simulink model "CoupledTanks_original"  (R2023b)
settings: Solver=ode45  StartTime=0.0  StopTime=400  MaxStep=1e-1  RelTol=1e-3  EnableMultiTasking=on
InitFcn:
  | g = 9.81; %gravitational constant
  | 
  | % showVR = 1; %show VR world
  | % h1_init = 0; %initial condition
  | % h2_init = 0; %initial condition
values from neighbouring files (symbols this model uses):
  K = place(Acl,Bcl, xd)    [ARI_SEM.m]
undefined symbols (not defined in the file or in its folder): P
libraries: vrlib x56, cstblocks x3, slpidlib x1
(part 1 of 2)
CloseFcn:
  | vrclose all;
  | clear figureVR worldVR;
settings Model: Creator=H  LastModifiedBy=pinki
settings SolverCC: AlgebraicLoopSolver=TrustRegion
settings DataIOCC: LimitDataPoints=on  SaveFormat=Array  SignalLoggingSaveFormat=ModelDataLogs  ReturnWorkspaceOutputs=off
settings OptimizationCC: ExpressionDepthLimit=2147483647  InitFltsAndDblsToZero=on  LifeSpan=inf
settings DebuggingCC: SaveWithParameterizedLinksMsg=none  UnderspecifiedInitializationDetection=Classic  MergeDetectMultiDrivingBlocksExec=none  SignalResolutionControl=TryResolveAllWithWarning  SolverPrmCheckMsg=warning  FcnCallInpInsideContextMsg=warning  UnconnectedInputMsg=warning  UnconnectedOutputMsg=warning  UnconnectedLineMsg=warning  StateNameClashWarn=warning  SFUnexpectedBacktrackingDiag=warning  SFNoUnconditionalDefaultTransitionDiag=warning  SFExecutionAtInitializationDiag=none  ArithmeticOperatorsInVariantConditions=warning
settings HardwareCC: ProdBitPerPointer=32  ProdBitPerSizeT=32  ProdBitPerPtrDiffT=32  ProdLargestAtomicFloat=None  ProdIntDivRoundTo=Undefined  ProdEndianess=Unspecified  ProdWordSize=32  ProdHWDeviceType=32-bit Generic
settings ModelReferenceCC: PropagateSignalLabelsOutOfModel=off
settings SFSimCC: SimUseLocalCustomCode=off  CustomCodeUndefinedFunction=UseInterfaceOnly
settings RTWCC: RTWUseLocalCustomCode=off
settings CodeAppCC: StateflowObjectComments=on
settings GRTTargetCC: TargetFcnLib=ansi_tfl_tmw.mat  TargetLangStandard=C89/C90 (ANSI)  CombineOutputUpdateFcns=off  GRTInterface=on
settings ConfigComp: CovMetricSettings=dw  CovSaveCumulativeToWorkspaceVar=on  CovSaveSingleToWorkspaceVar=on  CovExternalEMLEnable=off

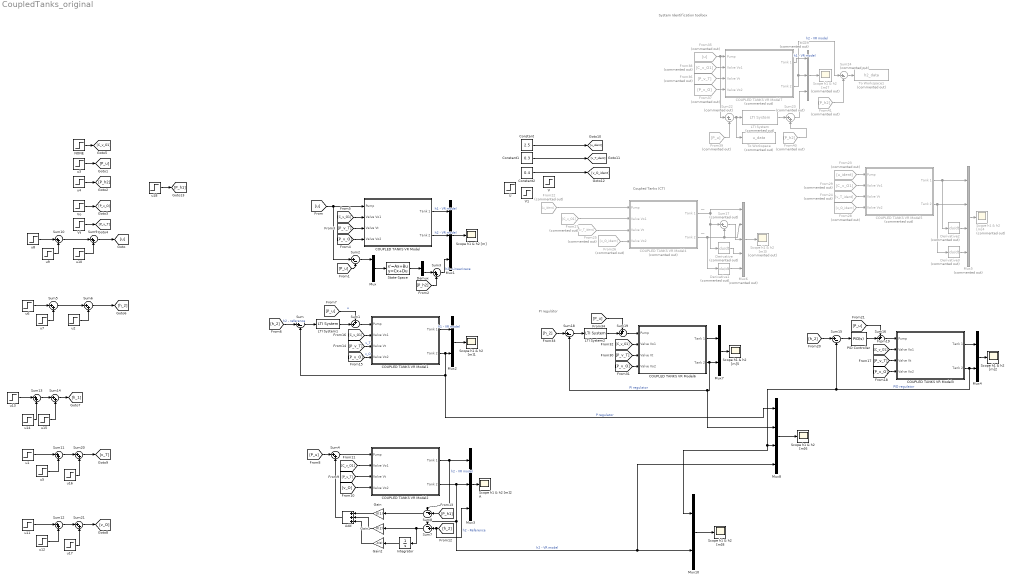
== system CoupledTanks_original ==
  note: System Identification toolbox
  note: PI regulátor
  note: __
  note: Coupled Tanks (CT)
  note: __
  Add : Sum  Inputs=+++
  COUPLED TANKS VR Model : Subsystem  mask(Coupled Tanks (CT) in laboratory K26){showVR=off, sfcnParam1=P.h1, sfcnParam2=P.h2}
      mask prompts: showVR "Show VirtualWorld?"; sfcnParam1 "Initial fluid level in the left tank 1   h1(0)  [cm]"; sfcnParam2 "Initial fluid  level in the right tank 2   h2 (0) [cm]"
      mask help:
      | Coupled Tanks (CT) in laboratory K26 - Virtual Reality
      | Real-Time Workshop generated S-function.
      mask Help:
      | Couple Tanks in laboratory K26 - Virtual Reality. <br><br>
      | 
      | 
      | This is a&nbsp;virtual model of the Coupled Tanks apparatus in Laboratory of automatic control
      | theory&nbsp;26 (<a href="http://support.dce.felk.cvut.cz/lab26/" target="_blank">http://support.dce.felk.cvut.cz/lab26/</a>),
      | which consists of a&nbsp;gear-pump, two tanks (left and right), inflow and outflow pipes and transfer (V<sub>t</sub>) and
      | output valves (V<sub>o1</sub>, V<sub>o2</sub>). The&nbsp;left tank is filled with the&nbsp;fluid by the&nbsp;gear-pump
      | controller by the&nbsp;voltage&nbsp;<em>u</em>&nbsp;[V]. The&nbsp;fluid can drain from the&nbsp;left tank through
      | the&nbsp;valve&nbsp;<em>v</em><sub>o1</sub>&nbsp;[%] or can drain to the&nbsp;right tank through the&nbsp;transfer
      | valve&nbsp;<em>v</em><sub>t</sub>&nbsp;[%]. The&nbsp;fluid drains away from the&nbsp;right tank through
      | the&nbsp;valve&nbsp;<em>v</em><sub>o2</sub>&nbsp;[%].<br><br>
      | 
      | The&nbsp;system input are the&nbsp;voltage of the&nbsp;motor of the&nbsp;gear-pump&nbsp;<em>u</em>&nbsp;[V]
      | and the&nbsp;opening of
      | the&nbsp;valves&nbsp;<em>v</em><sub>o1</sub>,&nbsp;<em>v</em><sub>t</sub>,&nbsp;<em>v</em><sub>o2</sub>&nbsp;[%].
      | The&nbsp;system outputs are the&nbsp;levels of the&nbsp;fluid in
      | the&nbsp;tanks&nbsp;<em>h</em><sub>1</sub>,&nbsp;<em>h</em><sub>2</sub>&nbsp;[cm].
      | The&nbsp;dynamics of the&nbsp;gear-pump is neglected. More information can be found on the&nbsp;website
      | <a href="http://support.dce.felk.cvut.cz/lab26/" target="_blank">http://support.dce.felk.cvut.cz/lab26/</a>.<br><br>
      | 
      | 
      | In the mask of the model, it can be set:
      | <ul>
      | <li>Initial fluid level in the left tank</li>
      | <li>Initial fluid level in the right tank.</li>
      | </ul><br><br>
      | 
      | 
      | Copyright: 2008, Jan Kricka, Jirka Roubal, Petr Husek.
      mask Callback showVR:
      | if strcmp('off',get_param(gcb,'showVR'))
      |     vrclose all;
      | else
      |     if exist('figureVR')==0
      |         figureVR = vrfigure;
      |     end
      |     if exist('worldVR')==0
      |         worldVR = vrworld('CoupledTanks_VR.WRL');
      |     end
      | 	if isvalid(figureVR)==0
      |         open(worldVR);
      |         figureVR = vrfigure(worldVR,[650 80 550 350]);
      | 	end
      | end
      mask Display:
      | image(imread('CoupledTanks_Image.jpg'));
      | port_label ('input',1,'u [V]');
      | port_label ('input',2,'Vo1 [-]');
      | port_label ('input',3,'Vt [-]');
      | port_label ('input',4,'Vo2 [-]');
      | port_label ('output',1,'h1 [m]');
      | port_label ('output',2,'h2 [m]');
  COUPLED TANKS VR Model1 : Subsystem  mask(Coupled Tanks (CT) in laboratory K26){showVR=off, sfcnParam1=P.h1, sfcnParam2=P.h2}
      mask prompts: showVR "Show VirtualWorld?"; sfcnParam1 "Initial fluid level in the left tank 1   h1(0)  [cm]"; sfcnParam2 "Initial fluid  level in the right tank 2   h2 (0) [cm]"
      mask help:
      | Coupled Tanks (CT) in laboratory K26 - Virtual Reality
      | Real-Time Workshop generated S-function.
      mask Help:
      | Couple Tanks in laboratory K26 - Virtual Reality. <br><br>
      | 
      | 
      | This is a&nbsp;virtual model of the Coupled Tanks apparatus in Laboratory of automatic control
      | theory&nbsp;26 (<a href="http://support.dce.felk.cvut.cz/lab26/" target="_blank">http://support.dce.felk.cvut.cz/lab26/</a>),
      | which consists of a&nbsp;gear-pump, two tanks (left and right), inflow and outflow pipes and transfer (V<sub>t</sub>) and
      | output valves (V<sub>o1</sub>, V<sub>o2</sub>). The&nbsp;left tank is filled with the&nbsp;fluid by the&nbsp;gear-pump
      | controller by the&nbsp;voltage&nbsp;<em>u</em>&nbsp;[V]. The&nbsp;fluid can drain from the&nbsp;left tank through
      | the&nbsp;valve&nbsp;<em>v</em><sub>o1</sub>&nbsp;[%] or can drain to the&nbsp;right tank through the&nbsp;transfer
      | valve&nbsp;<em>v</em><sub>t</sub>&nbsp;[%]. The&nbsp;fluid drains away from the&nbsp;right tank through
      | the&nbsp;valve&nbsp;<em>v</em><sub>o2</sub>&nbsp;[%].<br><br>
      | 
      | The&nbsp;system input are the&nbsp;voltage of the&nbsp;motor of the&nbsp;gear-pump&nbsp;<em>u</em>&nbsp;[V]
      | and the&nbsp;opening of
      | the&nbsp;valves&nbsp;<em>v</em><sub>o1</sub>,&nbsp;<em>v</em><sub>t</sub>,&nbsp;<em>v</em><sub>o2</sub>&nbsp;[%].
      | The&nbsp;system outputs are the&nbsp;levels of the&nbsp;fluid in
      | the&nbsp;tanks&nbsp;<em>h</em><sub>1</sub>,&nbsp;<em>h</em><sub>2</sub>&nbsp;[cm].
      | The&nbsp;dynamics of the&nbsp;gear-pump is neglected. More information can be found on the&nbsp;website
      | <a href="http://support.dce.felk.cvut.cz/lab26/" target="_blank">http://support.dce.felk.cvut.cz/lab26/</a>.<br><br>
      | 
      | 
      | In the mask of the model, it can be set:
      | <ul>
      | <li>Initial fluid level in the left tank</li>
      | <li>Initial fluid level in the right tank.</li>
      | </ul><br><br>
      | 
      | 
      | Copyright: 2008, Jan Kricka, Jirka Roubal, Petr Husek.
      mask Callback showVR:
      | if strcmp('off',get_param(gcb,'showVR'))
      |     vrclose all;
      | else
      |     if exist('figureVR')==0
      |         figureVR = vrfigure;
      |     end
      |     if exist('worldVR')==0
      |         worldVR = vrworld('CoupledTanks_VR.WRL');
      |     end
      | 	if isvalid(figureVR)==0
      |         open(worldVR);
      |         figureVR = vrfigure(worldVR,[650 80 550 350]);
      | 	end
      | end
      mask Display:
      | image(imread('CoupledTanks_Image.jpg'));
      | port_label ('input',1,'u [V]');
      | port_label ('input',2,'Vo1 [-]');
      | port_label ('input',3,'Vt [-]');
      | port_label ('input',4,'Vo2 [-]');
      | port_label ('output',1,'h1 [m]');
      | port_label ('output',2,'h2 [m]');
  COUPLED TANKS VR Model2 : Subsystem  mask(Coupled Tanks (CT) in laboratory K26){showVR=off, sfcnParam1=P.h1, sfcnParam2=P.h2}
      mask prompts: showVR "Show VirtualWorld?"; sfcnParam1 "Initial fluid level in the left tank 1   h1(0)  [cm]"; sfcnParam2 "Initial fluid  level in the right tank 2   h2 (0) [cm]"
      mask help:
      | Coupled Tanks (CT) in laboratory K26 - Virtual Reality
      | Real-Time Workshop generated S-function.
      mask Help:
      | Couple Tanks in laboratory K26 - Virtual Reality. <br><br>
      | 
      | 
      | This is a&nbsp;virtual model of the Coupled Tanks apparatus in Laboratory of automatic control
      | theory&nbsp;26 (<a href="http://support.dce.felk.cvut.cz/lab26/" target="_blank">http://support.dce.felk.cvut.cz/lab26/</a>),
      | which consists of a&nbsp;gear-pump, two tanks (left and right), inflow and outflow pipes and transfer (V<sub>t</sub>) and
      | output valves (V<sub>o1</sub>, V<sub>o2</sub>). The&nbsp;left tank is filled with the&nbsp;fluid by the&nbsp;gear-pump
      | controller by the&nbsp;voltage&nbsp;<em>u</em>&nbsp;[V]. The&nbsp;fluid can drain from the&nbsp;left tank through
      | the&nbsp;valve&nbsp;<em>v</em><sub>o1</sub>&nbsp;[%] or can drain to the&nbsp;right tank through the&nbsp;transfer
      | valve&nbsp;<em>v</em><sub>t</sub>&nbsp;[%]. The&nbsp;fluid drains away from the&nbsp;right tank through
      | the&nbsp;valve&nbsp;<em>v</em><sub>o2</sub>&nbsp;[%].<br><br>
      | 
      | The&nbsp;system input are the&nbsp;voltage of the&nbsp;motor of the&nbsp;gear-pump&nbsp;<em>u</em>&nbsp;[V]
      | and the&nbsp;opening of
      | the&nbsp;valves&nbsp;<em>v</em><sub>o1</sub>,&nbsp;<em>v</em><sub>t</sub>,&nbsp;<em>v</em><sub>o2</sub>&nbsp;[%].
      | The&nbsp;system outputs are the&nbsp;levels of the&nbsp;fluid in
      | the&nbsp;tanks&nbsp;<em>h</em><sub>1</sub>,&nbsp;<em>h</em><sub>2</sub>&nbsp;[cm].
      | The&nbsp;dynamics of the&nbsp;gear-pump is neglected. More information can be found on the&nbsp;website
      | <a href="http://support.dce.felk.cvut.cz/lab26/" target="_blank">http://support.dce.felk.cvut.cz/lab26/</a>.<br><br>
      | 
      | 
      | In the mask of the model, it can be set:
      | <ul>
      | <li>Initial fluid level in the left tank</li>
      | <li>Initial fluid level in the right tank.</li>
      | </ul><br><br>
      | 
      | 
      | Copyright: 2008, Jan Kricka, Jirka Roubal, Petr Husek.
      mask Callback showVR:
      | if strcmp('off',get_param(gcb,'showVR'))
      |     vrclose all;
      | else
      |     if exist('figureVR')==0
      |         figureVR = vrfigure;
      |     end
      |     if exist('worldVR')==0
      |         worldVR = vrworld('CoupledTanks_VR.WRL');
      |     end
      | 	if isvalid(figureVR)==0
      |         open(worldVR);
      |         figureVR = vrfigure(worldVR,[650 80 550 350]);
      | 	end
      | end
      mask Display:
      | image(imread('CoupledTanks_Image.jpg'));
      | port_label ('input',1,'u [V]');
      | port_label ('input',2,'Vo1 [-]');
      | port_label ('input',3,'Vt [-]');
      | port_label ('input',4,'Vo2 [-]');
      | port_label ('output',1,'h1 [m]');
      | port_label ('output',2,'h2 [m]');
  COUPLED TANKS VR Model3 : Subsystem  mask(Coupled Tanks (CT) in laboratory K26){showVR=off, sfcnParam1=P.h1, sfcnParam2=P.h2}
      mask prompts: showVR "Show VirtualWorld?"; sfcnParam1 "Initial fluid level in the left tank 1   h1(0)  [cm]"; sfcnParam2 "Initial fluid  level in the right tank 2   h2 (0) [cm]"
      mask help:
      | Coupled Tanks (CT) in laboratory K26 - Virtual Reality
      | Real-Time Workshop generated S-function.
      mask Help:
      | Couple Tanks in laboratory K26 - Virtual Reality. <br><br>
      | 
      | 
      | This is a&nbsp;virtual model of the Coupled Tanks apparatus in Laboratory of automatic control
      | theory&nbsp;26 (<a href="http://support.dce.felk.cvut.cz/lab26/" target="_blank">http://support.dce.felk.cvut.cz/lab26/</a>),
      | which consists of a&nbsp;gear-pump, two tanks (left and right), inflow and outflow pipes and transfer (V<sub>t</sub>) and
      | output valves (V<sub>o1</sub>, V<sub>o2</sub>). The&nbsp;left tank is filled with the&nbsp;fluid by the&nbsp;gear-pump
      | controller by the&nbsp;voltage&nbsp;<em>u</em>&nbsp;[V]. The&nbsp;fluid can drain from the&nbsp;left tank through
      | the&nbsp;valve&nbsp;<em>v</em><sub>o1</sub>&nbsp;[%] or can drain to the&nbsp;right tank through the&nbsp;transfer
      | valve&nbsp;<em>v</em><sub>t</sub>&nbsp;[%]. The&nbsp;fluid drains away from the&nbsp;right tank through
      | the&nbsp;valve&nbsp;<em>v</em><sub>o2</sub>&nbsp;[%].<br><br>
      | 
      | The&nbsp;system input are the&nbsp;voltage of the&nbsp;motor of the&nbsp;gear-pump&nbsp;<em>u</em>&nbsp;[V]
      | and the&nbsp;opening of
      | the&nbsp;valves&nbsp;<em>v</em><sub>o1</sub>,&nbsp;<em>v</em><sub>t</sub>,&nbsp;<em>v</em><sub>o2</sub>&nbsp;[%].
      | The&nbsp;system outputs are the&nbsp;levels of the&nbsp;fluid in
      | the&nbsp;tanks&nbsp;<em>h</em><sub>1</sub>,&nbsp;<em>h</em><sub>2</sub>&nbsp;[cm].
      | The&nbsp;dynamics of the&nbsp;gear-pump is neglected. More information can be found on the&nbsp;website
      | <a href="http://support.dce.felk.cvut.cz/lab26/" target="_blank">http://support.dce.felk.cvut.cz/lab26/</a>.<br><br>
      | 
      | 
      | In the mask of the model, it can be set:
      | <ul>
      | <li>Initial fluid level in the left tank</li>
      | <li>Initial fluid level in the right tank.</li>
      | </ul><br><br>
      | 
      | 
      | Copyright: 2008, Jan Kricka, Jirka Roubal, Petr Husek.
      mask Callback showVR:
      | if strcmp('off',get_param(gcb,'showVR'))
      |     vrclose all;
      | else
      |     if exist('figureVR')==0
      |         figureVR = vrfigure;
      |     end
      |     if exist('worldVR')==0
      |         worldVR = vrworld('CoupledTanks_VR.WRL');
      |     end
      | 	if isvalid(figureVR)==0
      |         open(worldVR);
      |         figureVR = vrfigure(worldVR,[650 80 550 350]);
      | 	end
      | end
      mask Display:
      | image(imread('CoupledTanks_Image.jpg'));
      | port_label ('input',1,'u [V]');
      | port_label ('input',2,'Vo1 [-]');
      | port_label ('input',3,'Vt [-]');
      | port_label ('input',4,'Vo2 [-]');
      | port_label ('output',1,'h1 [m]');
      | port_label ('output',2,'h2 [m]');
  COUPLED TANKS VR Model4 : Subsystem  Commented=on  mask(Coupled Tanks (CT) in laboratory K26){showVR=off, sfcnParam1=0, sfcnParam2=0}
      mask prompts: showVR "Show VirtualWorld?"; sfcnParam1 "Initial fluid level in the left tank 1   h1(0)  [cm]"; sfcnParam2 "Initial fluid  level in the right tank 2   h2 (0) [cm]"
      mask help:
      | Coupled Tanks (CT) in laboratory K26 - Virtual Reality
      | Real-Time Workshop generated S-function.
      mask Help:
      | Couple Tanks in laboratory K26 - Virtual Reality. <br><br>
      | 
      | 
      | This is a&nbsp;virtual model of the Coupled Tanks apparatus in Laboratory of automatic control
      | theory&nbsp;26 (<a href="http://support.dce.felk.cvut.cz/lab26/" target="_blank">http://support.dce.felk.cvut.cz/lab26/</a>),
      | which consists of a&nbsp;gear-pump, two tanks (left and right), inflow and outflow pipes and transfer (V<sub>t</sub>) and
      | output valves (V<sub>o1</sub>, V<sub>o2</sub>). The&nbsp;left tank is filled with the&nbsp;fluid by the&nbsp;gear-pump
      | controller by the&nbsp;voltage&nbsp;<em>u</em>&nbsp;[V]. The&nbsp;fluid can drain from the&nbsp;left tank through
      | the&nbsp;valve&nbsp;<em>v</em><sub>o1</sub>&nbsp;[%] or can drain to the&nbsp;right tank through the&nbsp;transfer
      | valve&nbsp;<em>v</em><sub>t</sub>&nbsp;[%]. The&nbsp;fluid drains away from the&nbsp;right tank through
      | the&nbsp;valve&nbsp;<em>v</em><sub>o2</sub>&nbsp;[%].<br><br>
      | 
      | The&nbsp;system input are the&nbsp;voltage of the&nbsp;motor of the&nbsp;gear-pump&nbsp;<em>u</em>&nbsp;[V]
      | and the&nbsp;opening of
      | the&nbsp;valves&nbsp;<em>v</em><sub>o1</sub>,&nbsp;<em>v</em><sub>t</sub>,&nbsp;<em>v</em><sub>o2</sub>&nbsp;[%].
      | The&nbsp;system outputs are the&nbsp;levels of the&nbsp;fluid in
      | the&nbsp;tanks&nbsp;<em>h</em><sub>1</sub>,&nbsp;<em>h</em><sub>2</sub>&nbsp;[cm].
      | The&nbsp;dynamics of the&nbsp;gear-pump is neglected. More information can be found on the&nbsp;website
      | <a href="http://support.dce.felk.cvut.cz/lab26/" target="_blank">http://support.dce.felk.cvut.cz/lab26/</a>.<br><br>
      | 
      | 
      | In the mask of the model, it can be set:
      | <ul>
      | <li>Initial fluid level in the left tank</li>
      | <li>Initial fluid level in the right tank.</li>
      | </ul><br><br>
      | 
      | 
      | Copyright: 2008, Jan Kricka, Jirka Roubal, Petr Husek.
      mask Callback showVR:
      | if strcmp('off',get_param(gcb,'showVR'))
      |     vrclose all;
      | else
      |     if exist('figureVR')==0
      |         figureVR = vrfigure;
      |     end
      |     if exist('worldVR')==0
      |         worldVR = vrworld('CoupledTanks_VR.WRL');
      |     end
      | 	if isvalid(figureVR)==0
      |         open(worldVR);
      |         figureVR = vrfigure(worldVR,[650 80 550 350]);
      | 	end
      | end
      mask Display:
      | image(imread('CoupledTanks_Image.jpg'));
      | port_label ('input',1,'u [V]');
      | port_label ('input',2,'Vo1 [-]');
      | port_label ('input',3,'Vt [-]');
      | port_label ('input',4,'Vo2 [-]');
      | port_label ('output',1,'h1 [m]');
      | port_label ('output',2,'h2 [m]');
  COUPLED TANKS VR Model5 : Subsystem  Commented=on  mask(Coupled Tanks (CT) in laboratory K26){showVR=off, sfcnParam1=0, sfcnParam2=0}
      mask prompts: showVR "Show VirtualWorld?"; sfcnParam1 "Initial fluid level in the left tank 1   h1(0)  [cm]"; sfcnParam2 "Initial fluid  level in the right tank 2   h2 (0) [cm]"
      mask help:
      | Coupled Tanks (CT) in laboratory K26 - Virtual Reality
      | Real-Time Workshop generated S-function.
      mask Help:
      | Couple Tanks in laboratory K26 - Virtual Reality. <br><br>
      | 
      | 
      | This is a&nbsp;virtual model of the Coupled Tanks apparatus in Laboratory of automatic control
      | theory&nbsp;26 (<a href="http://support.dce.felk.cvut.cz/lab26/" target="_blank">http://support.dce.felk.cvut.cz/lab26/</a>),
      | which consists of a&nbsp;gear-pump, two tanks (left and right), inflow and outflow pipes and transfer (V<sub>t</sub>) and
      | output valves (V<sub>o1</sub>, V<sub>o2</sub>). The&nbsp;left tank is filled with the&nbsp;fluid by the&nbsp;gear-pump
      | controller by the&nbsp;voltage&nbsp;<em>u</em>&nbsp;[V]. The&nbsp;fluid can drain from the&nbsp;left tank through
      | the&nbsp;valve&nbsp;<em>v</em><sub>o1</sub>&nbsp;[%] or can drain to the&nbsp;right tank through the&nbsp;transfer
      | valve&nbsp;<em>v</em><sub>t</sub>&nbsp;[%]. The&nbsp;fluid drains away from the&nbsp;right tank through
      | the&nbsp;valve&nbsp;<em>v</em><sub>o2</sub>&nbsp;[%].<br><br>
      | 
      | The&nbsp;system input are the&nbsp;voltage of the&nbsp;motor of the&nbsp;gear-pump&nbsp;<em>u</em>&nbsp;[V]
      | and the&nbsp;opening of
      | the&nbsp;valves&nbsp;<em>v</em><sub>o1</sub>,&nbsp;<em>v</em><sub>t</sub>,&nbsp;<em>v</em><sub>o2</sub>&nbsp;[%].
      | The&nbsp;system outputs are the&nbsp;levels of the&nbsp;fluid in
      | the&nbsp;tanks&nbsp;<em>h</em><sub>1</sub>,&nbsp;<em>h</em><sub>2</sub>&nbsp;[cm].
      | The&nbsp;dynamics of the&nbsp;gear-pump is neglected. More information can be found on the&nbsp;website
      | <a href="http://support.dce.felk.cvut.cz/lab26/" target="_blank">http://support.dce.felk.cvut.cz/lab26/</a>.<br><br>
      | 
      | 
      | In the mask of the model, it can be set:
      | <ul>
      | <li>Initial fluid level in the left tank</li>
      | <li>Initial fluid level in the right tank.</li>
      | </ul><br><br>
      | 
      | 
      | Copyright: 2008, Jan Kricka, Jirka Roubal, Petr Husek.
      mask Callback showVR:
      | if strcmp('off',get_param(gcb,'showVR'))
      |     vrclose all;
      | else
      |     if exist('figureVR')==0
      |         figureVR = vrfigure;
      |     end
      |     if exist('worldVR')==0
      |         worldVR = vrworld('CoupledTanks_VR.WRL');
      |     end
      | 	if isvalid(figureVR)==0
      |         open(worldVR);
      |         figureVR = vrfigure(worldVR,[650 80 550 350]);
      | 	end
      | end
      mask Display:
      | image(imread('CoupledTanks_Image.jpg'));
      | port_label ('input',1,'u [V]');
      | port_label ('input',2,'Vo1 [-]');
      | port_label ('input',3,'Vt [-]');
      | port_label ('input',4,'Vo2 [-]');
      | port_label ('output',1,'h1 [m]');
      | port_label ('output',2,'h2 [m]');
  COUPLED TANKS VR Model6 : Subsystem  mask(Coupled Tanks (CT) in laboratory K26){showVR=off, sfcnParam1=P.h1, sfcnParam2=P.h2}
      mask prompts: showVR "Show VirtualWorld?"; sfcnParam1 "Initial fluid level in the left tank 1   h1(0)  [cm]"; sfcnParam2 "Initial fluid  level in the right tank 2   h2 (0) [cm]"
      mask help:
      | Coupled Tanks (CT) in laboratory K26 - Virtual Reality
      | Real-Time Workshop generated S-function.
      mask Help:
      | Couple Tanks in laboratory K26 - Virtual Reality. <br><br>
      | 
      | 
      | This is a&nbsp;virtual model of the Coupled Tanks apparatus in Laboratory of automatic control
      | theory&nbsp;26 (<a href="http://support.dce.felk.cvut.cz/lab26/" target="_blank">http://support.dce.felk.cvut.cz/lab26/</a>),
      | which consists of a&nbsp;gear-pump, two tanks (left and right), inflow and outflow pipes and transfer (V<sub>t</sub>) and
      | output valves (V<sub>o1</sub>, V<sub>o2</sub>). The&nbsp;left tank is filled with the&nbsp;fluid by the&nbsp;gear-pump
      | controller by the&nbsp;voltage&nbsp;<em>u</em>&nbsp;[V]. The&nbsp;fluid can drain from the&nbsp;left tank through
      | the&nbsp;valve&nbsp;<em>v</em><sub>o1</sub>&nbsp;[%] or can drain to the&nbsp;right tank through the&nbsp;transfer
      | valve&nbsp;<em>v</em><sub>t</sub>&nbsp;[%]. The&nbsp;fluid drains away from the&nbsp;right tank through
      | the&nbsp;valve&nbsp;<em>v</em><sub>o2</sub>&nbsp;[%].<br><br>
      | 
      | The&nbsp;system input are the&nbsp;voltage of the&nbsp;motor of the&nbsp;gear-pump&nbsp;<em>u</em>&nbsp;[V]
      | and the&nbsp;opening of
      | the&nbsp;valves&nbsp;<em>v</em><sub>o1</sub>,&nbsp;<em>v</em><sub>t</sub>,&nbsp;<em>v</em><sub>o2</sub>&nbsp;[%].
      | The&nbsp;system outputs are the&nbsp;levels of the&nbsp;fluid in
      | the&nbsp;tanks&nbsp;<em>h</em><sub>1</sub>,&nbsp;<em>h</em><sub>2</sub>&nbsp;[cm].
      | The&nbsp;dynamics of the&nbsp;gear-pump is neglected. More information can be found on the&nbsp;website
      | <a href="http://support.dce.felk.cvut.cz/lab26/" target="_blank">http://support.dce.felk.cvut.cz/lab26/</a>.<br><br>
      | 
      | 
      | In the mask of the model, it can be set:
      | <ul>
      | <li>Initial fluid level in the left tank</li>
      | <li>Initial fluid level in the right tank.</li>
      | </ul><br><br>
      | 
      | 
      | Copyright: 2008, Jan Kricka, Jirka Roubal, Petr Husek.
      mask Callback showVR:
      | if strcmp('off',get_param(gcb,'showVR'))
      |     vrclose all;
      | else
      |     if exist('figureVR')==0
      |         figureVR = vrfigure;
      |     end
      |     if exist('worldVR')==0
      |         worldVR = vrworld('CoupledTanks_VR.WRL');
      |     end
      | 	if isvalid(figureVR)==0
      |         open(worldVR);
      |         figureVR = vrfigure(worldVR,[650 80 550 350]);
      | 	end
      | end
      mask Display:
      | image(imread('CoupledTanks_Image.jpg'));
      | port_label ('input',1,'u [V]');
      | port_label ('input',2,'Vo1 [-]');
      | port_label ('input',3,'Vt [-]');
      | port_label ('input',4,'Vo2 [-]');
      | port_label ('output',1,'h1 [m]');
      | port_label ('output',2,'h2 [m]');
  COUPLED TANKS VR Model7 : Subsystem  Commented=on  mask(Coupled Tanks (CT) in laboratory K26){showVR=off, sfcnParam1=P.h1, sfcnParam2=P.h2}
      mask prompts: showVR "Show VirtualWorld?"; sfcnParam1 "Initial fluid level in the left tank 1   h1(0)  [cm]"; sfcnParam2 "Initial fluid  level in the right tank 2   h2 (0) [cm]"
      mask help:
      | Coupled Tanks (CT) in laboratory K26 - Virtual Reality
      | Real-Time Workshop generated S-function.
      mask Help:
      | Couple Tanks in laboratory K26 - Virtual Reality. <br><br>
      | 
      | 
      | This is a&nbsp;virtual model of the Coupled Tanks apparatus in Laboratory of automatic control
      | theory&nbsp;26 (<a href="http://support.dce.felk.cvut.cz/lab26/" target="_blank">http://support.dce.felk.cvut.cz/lab26/</a>),
      | which consists of a&nbsp;gear-pump, two tanks (left and right), inflow and outflow pipes and transfer (V<sub>t</sub>) and
      | output valves (V<sub>o1</sub>, V<sub>o2</sub>). The&nbsp;left tank is filled with the&nbsp;fluid by the&nbsp;gear-pump
      | controller by the&nbsp;voltage&nbsp;<em>u</em>&nbsp;[V]. The&nbsp;fluid can drain from the&nbsp;left tank through
      | the&nbsp;valve&nbsp;<em>v</em><sub>o1</sub>&nbsp;[%] or can drain to the&nbsp;right tank through the&nbsp;transfer
      | valve&nbsp;<em>v</em><sub>t</sub>&nbsp;[%]. The&nbsp;fluid drains away from the&nbsp;right tank through
      | the&nbsp;valve&nbsp;<em>v</em><sub>o2</sub>&nbsp;[%].<br><br>
      | 
      | The&nbsp;system input are the&nbsp;voltage of the&nbsp;motor of the&nbsp;gear-pump&nbsp;<em>u</em>&nbsp;[V]
      | and the&nbsp;opening of
      | the&nbsp;valves&nbsp;<em>v</em><sub>o1</sub>,&nbsp;<em>v</em><sub>t</sub>,&nbsp;<em>v</em><sub>o2</sub>&nbsp;[%].
      | The&nbsp;system outputs are the&nbsp;levels of the&nbsp;fluid in
      | the&nbsp;tanks&nbsp;<em>h</em><sub>1</sub>,&nbsp;<em>h</em><sub>2</sub>&nbsp;[cm].
      | The&nbsp;dynamics of the&nbsp;gear-pump is neglected. More information can be found on the&nbsp;website
      | <a href="http://support.dce.felk.cvut.cz/lab26/" target="_blank">http://support.dce.felk.cvut.cz/lab26/</a>.<br><br>
      | 
      | 
      | In the mask of the model, it can be set:
      | <ul>
      | <li>Initial fluid level in the left tank</li>
      | <li>Initial fluid level in the right tank.</li>
      | </ul><br><br>
      | 
      | 
      | Copyright: 2008, Jan Kricka, Jirka Roubal, Petr Husek.
      mask Callback showVR:
      | if strcmp('off',get_param(gcb,'showVR'))
      |     vrclose all;
      | else
      |     if exist('figureVR')==0
      |         figureVR = vrfigure;
      |     end
      |     if exist('worldVR')==0
      |         worldVR = vrworld('CoupledTanks_VR.WRL');
      |     end
      | 	if isvalid(figureVR)==0
      |         open(worldVR);
      |         figureVR = vrfigure(worldVR,[650 80 550 350]);
      | 	end
      | end
      mask Display:
      | image(imread('CoupledTanks_Image.jpg'));
      | port_label ('input',1,'u [V]');
      | port_label ('input',2,'Vo1 [-]');
      | port_label ('input',3,'Vt [-]');
      | port_label ('input',4,'Vo2 [-]');
      | port_label ('output',1,'h1 [m]');
      | port_label ('output',2,'h2 [m]');
  Constant : Constant  Value=2.5
  Constant1 : Constant  Value=0.3
  Constant2 : Constant  Value=0.4
  Demux : Demux  Outputs=2
  Derivative{,1..3} (4 alike) : Derivative  Commented=on
  From22 : From  Commented=on  GotoTag=u_ident
  From23 : From  Commented=on  GotoTag=u_ident
  From24 : From  Commented=on  GotoTag=v_T_ident
  From25 : From  Commented=on  GotoTag=v_T_ident
  From26 : From  Commented=on  GotoTag=v_O_ident
  From27 : From  Commented=on  GotoTag=C_v_O1
  From28 : From  Commented=on  GotoTag=v_O_ident
  From29 : From  Commented=on  GotoTag=C_v_O1
  From35 : From  Commented=on  GotoTag=u
  From36 : From  Commented=on  GotoTag=P_v_T
  From37 : From  Commented=on  GotoTag=P_v_O
  From38 : From  Commented=on  GotoTag=C_v_O1
  From39 : From  Commented=on  GotoTag=P_u
  From40 : From  Commented=on  GotoTag=P_h2
  From41 : From  Commented=on  GotoTag=P_h2
  Gain : Gain  Gain=K(1)
  Gain1 : Gain  Gain=K(2)
  Gain2 : Gain  Gain=-K(3)
  Integrator : Integrator
  LTI System : cstblocks/LTI System  Commented=on  sys=tf7  IC=[]  PadeOrder=0
  LTI System1 : cstblocks/LTI System  sys=SISO_P  IC=[0.2025,0.135]  PadeOrder=0
  LTI System2 : cstblocks/LTI System  sys=C_RL_PI  IC=[0.2025,0.135]  PadeOrder=0
  Mux : Mux  Inputs=3
  Mux1 : Mux  Inputs=3
  Mux{2,4,7,10} (4 alike) : Mux  Inputs=2
  Mux3 : Mux  Inputs=3
  Mux5 : Mux  Commented=on
  Mux6 : Mux  Commented=on  Inputs=5
  Mux8 : Mux
  Mux9 : Mux  Commented=on  Inputs=3
  NONE : Step  Time=0  After=0  SampleTime=0
  PID Controller : slpidlib/PID Controller  Controller=PID  Form=Parallel  TimeDomain=Continuous-time  UseExternalTs=off  SampleTime=-1  IntegratorMethod=Forward Euler  FilterMethod=Forward Euler  ControllerParametersSource=internal  P=820.310009598714  I=206.957781528815  UseKiTs=off  D=583.23832095892  N=6.74685229285638  UseFilter=on  TunerSelectOption=Transfer Function Based (PID Tuner App)  InitialConditionSource=internal  InitialConditionForIntegrator=0  InitialConditionForFilter=0  DifferentiatorICPrevScaledInput=0  ExternalReset=none  TrackingMode=off  Kt=1  LimitOutput=off  SatLimitsSource=internal  UpperSaturationLimit=inf  LowerSaturationLimit=-inf  LinearizeAsGain=on  AntiWindupMode=none  Kb=1  LimitIntegrator=off  UpperIntegratorSaturationLimit=inf  LowerIntegratorSaturationLimit=-inf  POutMin=[]  POutMax=[]  IOutMin=[]  IOutMax=[]  DOutMin=[]  DOutMax=[]  NOutMin=[]  NOutMax=[]  SumOutMin=[]  SumOutMax=[]  SaturationOutMin=[]  SaturationOutMax=[]  PParamMin=[]  PParamMax=[]  IParamMin=[]  IParamMax=[]  DParamMin=[]  DParamMax=[]  NParamMin=[]  NParamMax=[]  KbParamMin=[]  KbParamMax=[]  KtParamMin=[]  KtParamMax=[]  KbOutMin=[]  KbOutMax=[]  KtOutMin=[]  KtOutMax=[]  IntegratorOutMin=[]  IntegratorOutMax=[]  FilterOutMin=[]  FilterOutMax=[]  SumI1OutMin=[]  SumI1OutMax=[]  SumI2OutMin=[]  SumI2OutMax=[]  SumI3OutMin=[]  SumI3OutMax=[]  SumI4OutMin=[]  SumI4OutMax=[]  SumDOutMin=[]  SumDOutMax=[]  DifferentiatorOutMin=[]  DifferentiatorOutMax=[]  FilterDiffOutCoefMin=[]  FilterDiffOutCoefMax=[]  ReciprocalOutMin=[]  ReciprocalOutMax=[]  SumDenOutMin=[]  SumDenOutMax=[]  SumNumOutMin=[]  SumNumOutMax=[]  DivideOutMin=[]  DivideOutMax=[]  UdiffTsProdOutMin=[]  UdiffTsProdOutMax=[]  NTsProdOutMin=[]  NTsProdOutMax=[]  UintegralTsProdOutMin=[]  UintegralTsProdOutMax=[]  UngainTsProdOutMin=[]  UngainTsProdOutMax=[]  ClampingZeroOutDataTypeStr=Inherit: Inherit via back propagation  ClampingZeroOutMin=[]  ClampingZeroOutMax=[]  FilterDenConstantOutDataTypeStr=Inherit: Inherit via back propagation  FilterDenConstantOutMin=[]  FilterDenConstantOutMax=[]  PCopyOutDataTypeStr=Inherit: Inherit via back propagation  PCopyOutMin=[]  PCopyOutMax=[]  NCopyOutDataTypeStr=Inherit: Inherit via back propagation  NCopyOutMin=[]  NCopyOutMax=[]  IntegratorContinuousStateAttributes=''  IntegratorStateMustResolveToSignalObject=off  IntegratorRTWStateStorageClass=Auto  FilterContinuousStateAttributes=''  FilterStateMustResolveToSignalObject=off  FilterRTWStateStorageClass=Auto  ParallelPVariant=InternalParameters  IdealPVariant=Disabled  IVariant=InternalParameters  DVariant=InternalParameters  IntegratorVariant=Continuous  SatVariant=Disabled  AWVariant=Passthrough  PCopyVariant=Disabled  TRVariant=Disabled  FdbkBlocksVariant=Forward  IdealPFdbkVariant=Disabled  SatFdbkVariant=Disabled  DerivativeFilterVariant=ContFilter  NVariant=InternalParameters  NCopyVariant=Disabled  FilterICVariant=InternalICsFilter  IntegratorICVariant=InternalICs  ExternalResetVariant=Disabled  TRSumVariant=Passthrough  SumFdbkVariant=Disabled  SumVariant=Sum_PID  TsampFilterVariant=InternalTs  TsampNgainVariant=Passthrough  TsampIntegralVariant=Disabled_SignalSpec  ExternalSaturationOutDataTypeStr=Inherit: Same as second input
  Scope h1 & h2 [m]{,1..2,5..6,8} (6 alike) : Scope
  Scope h1 & h2 [m]2 A : Scope
  Scope h1 & h2 [m]3 : Scope  Commented=on
  Scope h1 & h2 [m]4 : Scope  Commented=on
  Scope h1 & h2 [m]7 : Scope  Commented=on
  State-Space : StateSpace  A=P.A  B=P.B  C=P.C  D=P.D  InitialCondition=0
  Sum{,2,15,18} (4 alike) : Sum  Inputs=|+-
  Sum1 : Sum  Inputs=++|
  Sum{3..6,9..14,20..21} (12 alike) : Sum  Inputs=|++
  Sum16 : Sum  Inputs=++|
  Sum17 : Sum  Commented=on  Inputs=|+-
  Sum19 : Sum  Inputs=++|
  Sum22 : Sum  Commented=on  Inputs=|+-
  Sum23 : Sum  Commented=on  Inputs=|++
  Sum24 : Sum  Commented=on  Inputs=|+-
  Sum7 : Sum  Inputs=-+|
  Sum8 : Sum  Inputs=-+|
  To Workspace : ToWorkspace  Commented=on  VariableName=u_data  SampleTime=-1
  To Workspace1 : ToWorkspace  Commented=on  VariableName=h2_data  SampleTime=-1
  U : Step  Time=100  Before=1  After=0  SampleTime=0
  V : Step  Time=100  SampleTime=0
  V1 : Step  Time=100  SampleTime=0
  Vo : Step  Time=0  Before=0.3  After=0.3  SampleTime=0
  Vt : Step  Time=0  Before=0.4  After=0.4  SampleTime=0
  u1 : Step  Time=100  Before=P.v_T  After=P.v_T+0.1  SampleTime=0
  u10 : Step  Time=300  After=2  SampleTime=0
  u11 : Step  Time=100  Before=P.v_O  After=P.v_O+0.1  SampleTime=0
  u12 : Step  Time=200  After=-0.2  SampleTime=0
  u13 : Step  Time=100  Before=P.h1  After=P.h1+0.005  SampleTime=0
  u14 : Step  Time=200  After=-0.01  SampleTime=0
  u15 : Step  Time=300  After=0.015  SampleTime=0
  u16 : Step  Time=300  After=0.4  SampleTime=0
  u17 : Step  Time=300  After=0.4  SampleTime=0
  u18 : Step  Time=0  Before=P.h1  After=P.h1  SampleTime=0
  u2 : Step  Time=300  After=0.02  SampleTime=0
  u3 : Step  Time=0  Before=P.u  After=P.u  SampleTime=0
  u4 : Step  Time=0  Before=P.h2  After=P.h2  SampleTime=0
  u5 : Step  Time=200  After=-0.2  SampleTime=0
  u6 : Step  Time=100  Before=P.h2  After=P.h2+0.005  SampleTime=0
  u7 : Step  Time=200  After=-0.01  SampleTime=0
  u8 : Step  Time=100  Before=P.u  After=P.u+0.5  SampleTime=0
  u9 : Step  Time=200  After=-1  SampleTime=0
  wires:
  Mux1/1 -> Scope h1 & h2 [m]/1
  Mux2/1 -> Scope h1 & h2 [m]1/1
  COUPLED TANKS VR Model1/2(Tank 2) -> Mux8/1, Sum/2, Mux2/2  "P regulator"
  COUPLED TANKS VR Model1/1(Tank 1) -> Mux2/1  "h1 - VR model"
  Sum1/1 -> COUPLED TANKS VR Model1/1(Pump)
  Sum3/1 -> Mux1/3  "h2 - Linearizace"
  Mux/1 -> State-Space/1
  Sum2/1 -> Mux/1
  State-Space/1 -> Demux/1
  Demux/2 -> Sum3/1
  COUPLED TANKS VR Model/1(Tank 1) -> Mux1/1  "h1 - VR model"
  COUPLED TANKS VR Model/2(Tank 2) -> Mux1/2  "h2 - VR model"
  [P_v_T] -> COUPLED TANKS VR Model2/3(Valve Vt)
  [C_v_O1] -> COUPLED TANKS VR Model2/2(Valve Vo1)
  Sum4/1 -> COUPLED TANKS VR Model2/1(Pump)
  COUPLED TANKS VR Model2/2(Tank 2) -> Mux8/4, Mux10/2, Sum7/1, Mux3/2  "h2 - VR model"
  [P_u] -> Sum4/1
  Mux3/1 -> Scope h1 & h2 [m]2 A/1
  COUPLED TANKS VR Model2/1(Tank 1) -> Sum8/1, Mux3/1  "h2 - VR model"
  [P_u] -> Sum1/1  "u"
  Integrator/1 -> Gain2/1
  Gain1/1 -> Add/2
  Gain/1 -> Add/1
  Gain2/1 -> Add/3
  Sum8/1 -> Gain/1
  Sum7/1 -> Integrator/1, Gain1/1
  [P_h1] -> Sum8/2
  [h_2] -> Mux3/3, Sum7/2  "h2 - Reference"
  Add/1 -> Sum4/2
  u8/1 -> Sum10/1
  u10/1 -> Sum9/2
  Sum10/1 -> Sum9/1
  u9/1 -> Sum10/2
  Sum9/1 -> [u]
  [u] -> Sum2/1, COUPLED TANKS VR Model/1(Pump)
  u3/1 -> [P_u]
  [P_u] -> Sum2/2
  u4/1 -> [P_h2]
  [P_h2] -> Sum3/2
  Vo/1 -> [P_v_O]
  [P_v_O] -> COUPLED TANKS VR Model/4(Valve Vo2)
  Vt/1 -> [P_v_T]
  [P_v_T] -> COUPLED TANKS VR Model/3(Valve Vt)
  NONE/1 -> [C_v_O1]
  [C_v_O1] -> COUPLED TANKS VR Model/2(Valve Vo1)
  [h_2] -> Sum/1  "h2 - reference"
  u2/1 -> Sum6/2
  Sum5/1 -> Sum6/1
  u7/1 -> Sum5/2
  Sum6/1 -> [h_2]
  u6/1 -> Sum5/1
  [v_O] -> COUPLED TANKS VR Model2/4(Valve Vo2)
  u1/1 -> Sum11/1
  u5/1 -> Sum11/2
  u12/1 -> Sum12/2
  u11/1 -> Sum12/1
  [P_v_T] -> COUPLED TANKS VR Model1/3(Valve Vt)  "v_T"
  [C_v_O1] -> COUPLED TANKS VR Model1/2(Valve Vo1)
  [P_v_O] -> COUPLED TANKS VR Model1/4(Valve Vo2)  "v_O"
  u13/1 -> Sum13/1
  u14/1 -> Sum13/2
  Sum14/1 -> [h_1]
  Sum13/1 -> Sum14/1
  u15/1 -> Sum14/2
  PID Controller/1 -> Sum16/2
  COUPLED TANKS VR Model3/2(Tank 2) -> Mux10/1, Mux8/3, Sum15/2, Mux4/2  "PID regulator"
  Sum15/1 -> PID Controller/1
  COUPLED TANKS VR Model3/1(Tank 1) -> Mux4/1
  Mux4/1 -> Scope h1 & h2 [m]2/1
  [P_v_T] -> COUPLED TANKS VR Model3/3(Valve Vt)
  Sum16/1 -> COUPLED TANKS VR Model3/1(Pump)
  [P_u] -> Sum16/1
  [h_2] -> Sum15/1
  [P_v_O] -> COUPLED TANKS VR Model3/4(Valve Vo2)
  [C_v_O1] -> COUPLED TANKS VR Model3/2(Valve Vo1)
  Mux6/1 -> Scope h1 & h2 [m]3/1
  COUPLED TANKS VR Model4/1(Tank 1) -> Derivative/1, Sum17/1, Mux6/1
  COUPLED TANKS VR Model4/2(Tank 2) -> Sum17/2, Mux6/2, Derivative1/1
  From26/1 -> COUPLED TANKS VR Model4/4(Valve Vo2)
  From25/1 -> COUPLED TANKS VR Model4/3(Valve Vt)
  From27/1 -> COUPLED TANKS VR Model4/2(Valve Vo1)
  From22/1 -> COUPLED TANKS VR Model4/1(Pump)
  Sum17/1 -> Mux6/3
  Derivative/1 -> Mux6/4
  Derivative1/1 -> Mux6/5
  Constant2/1 -> [v_O_ident]
  Constant1/1 -> [v_T_ident]
  Constant/1 -> [u_ident]
  From23/1 -> COUPLED TANKS VR Model5/1(Pump)
  Mux5/1 -> Scope h1 & h2 [m]4/1
  From29/1 -> COUPLED TANKS VR Model5/2(Valve Vo1)
  From24/1 -> COUPLED TANKS VR Model5/3(Valve Vt)
  From28/1 -> COUPLED TANKS VR Model5/4(Valve Vo2)
  COUPLED TANKS VR Model5/1(Tank 1) -> Mux5/1, Derivative2/1
  COUPLED TANKS VR Model5/2(Tank 2) -> Mux5/2, Derivative3/1
  Derivative2/1 -> Mux5/3
  Derivative3/1 -> Mux5/4
  Sum19/1 -> COUPLED TANKS VR Model6/1(Pump)
  [P_v_T] -> COUPLED TANKS VR Model6/3(Valve Vt)
  [P_v_O] -> COUPLED TANKS VR Model6/4(Valve Vo2)
  [h_2] -> Sum18/1
  [C_v_O1] -> COUPLED TANKS VR Model6/2(Valve Vo1)
  [P_u] -> Sum19/1
  COUPLED TANKS VR Model6/2(Tank 2) -> Mux8/2, Sum18/2, Mux7/2  "PI regulator"
  COUPLED TANKS VR Model6/1(Tank 1) -> Mux7/1
  Sum18/1 -> LTI System2/1
  Mux7/1 -> Scope h1 & h2 [m]5/1
  LTI System2/1 -> Sum19/2
  Mux8/1 -> Scope h1 & h2 [m]6/1
  u16/1 -> Sum20/2
  Sum11/1 -> Sum20/1
  Sum20/1 -> [v_T]
  Sum12/1 -> Sum21/1
  Sum21/1 -> [v_O]
  u17/1 -> Sum21/2
  LTI System1/1 -> Sum1/2
  Sum/1 -> LTI System1/1
  COUPLED TANKS VR Model7/2(Tank 2) -> Sum24/1, Mux9/2  "h2 - VR model"
  From38/1 -> COUPLED TANKS VR Model7/2(Valve Vo1)
  COUPLED TANKS VR Model7/1(Tank 1) -> Mux9/1  "h1 - VR model"
  From37/1 -> COUPLED TANKS VR Model7/4(Valve Vo2)
  Mux9/1 -> Scope h1 & h2 [m]7/1
  From36/1 -> COUPLED TANKS VR Model7/3(Valve Vt)
  Sum22/1 -> To Workspace/1, LTI System/1
  LTI System/1 -> Sum23/1
  From35/1 -> Sum22/1, COUPLED TANKS VR Model7/1(Pump)
  From39/1 -> Sum22/2
  From40/1 -> Sum23/2
  Sum23/1 -> Mux9/3
  From41/1 -> Sum24/2
  Sum24/1 -> To Workspace1/1
  u18/1 -> [P_h1]
  Mux10/1 -> Scope h1 & h2 [m]8/1

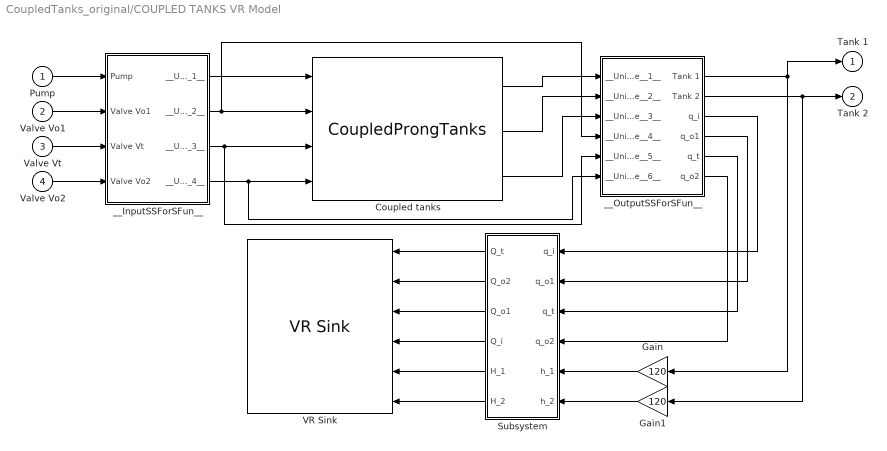
== system CoupledTanks_original/COUPLED TANKS VR Model ==
  Pump : Inport
  Valve Vo1 : Inport  Port=2
  Valve Vt : Inport  Port=3
  Valve Vo2 : Inport  Port=4
  Coupled tanks : M-S-Function  FunctionName=CoupledProngTanks  Parameters=h10 h20  mask{h10=sfcnParam1, h20=sfcnParam2}
      mask prompts: h10 "h1_init"; h20 "h2_init"
      mask Display:
      | port_label('input',1,'Pump');
      | port_label('input',2,'Valve Vo1');
      | port_label('input',3,'Valve Vt');
      | port_label('input',4,'Valve Vo2');
      | port_label('output',1,'Tank 1');
      | port_label('output',2,'Tank 2');
      | port_label('output',3,'q_i');
  Gain : Gain  Gain=120
  Gain1 : Gain  Gain=120
  Subsystem : Subsystem
  VR Sink : vrlib/VR Sink  InstantiateOnLoad=on  SampleTime=-1  ViewEnable=on  RemoteChange=off  RemoteView=on  FieldsWritten=Valve_t.rotation.4.1.double#Valve_o2.rotation.4.1.double#Valve_o1.rotation.4.1.double#Pump.rotation.4.1.double#water1.scale.3.1.double#water2.scale.3.1.double  WorldFileName=CoupledTanks_VR.WRL  AutoView=off  VideoDimensions=[]  AllowVariableSize=off
  __InputSSForSFun__ : Subsystem
  __OutputSSForSFun__ : Subsystem
  Tank 1 : Outport  OutDataTypeStr=double  PortDimensions=1  SampleTime=[-1 0]
  Tank 2 : Outport  Port=2  OutDataTypeStr=double  PortDimensions=1  SampleTime=[-1 0]
  wires:
  __OutputSSForSFun__/6(q_o2) -> Subsystem/4(q_o2)
  __OutputSSForSFun__/5(q_t) -> Subsystem/3(q_t)
  __OutputSSForSFun__/4(q_o1) -> Subsystem/2(q_o1)
  __OutputSSForSFun__/3(q_i) -> Subsystem/1(q_i)
  Subsystem/2(Q_o2) -> VR Sink/2
  Subsystem/3(Q_o1) -> VR Sink/3
  Subsystem/4(Q_i) -> VR Sink/4
  Subsystem/1(Q_t) -> VR Sink/1
  Subsystem/6(H_2) -> VR Sink/6
  Subsystem/5(H_1) -> VR Sink/5
  __OutputSSForSFun__/2(Tank 2) -> Gain1/1, Tank 2/1
  __OutputSSForSFun__/1(Tank 1) -> Tank 1/1, Gain/1
  __InputSSForSFun__/4(__UniqueOutportName__4__) -> __OutputSSForSFun__/6(__UniqueInportName__6__), Coupled tanks/4
  __InputSSForSFun__/3(__UniqueOutportName__3__) -> __OutputSSForSFun__/5(__UniqueInportName__5__), Coupled tanks/3
  Coupled tanks/2 -> __OutputSSForSFun__/2(__UniqueInportName__2__)
  Coupled tanks/1 -> __OutputSSForSFun__/1(__UniqueInportName__1__)
  __InputSSForSFun__/2(__UniqueOutportName__2__) -> __OutputSSForSFun__/4(__UniqueInportName__4__), Coupled tanks/2
  __InputSSForSFun__/1(__UniqueOutportName__1__) -> Coupled tanks/1
  Valve Vo2/1 -> __InputSSForSFun__/4(Valve Vo2)
  Valve Vt/1 -> __InputSSForSFun__/3(Valve Vt)
  Valve Vo1/1 -> __InputSSForSFun__/2(Valve Vo1)
  Pump/1 -> __InputSSForSFun__/1(Pump)
  Coupled tanks/3 -> __OutputSSForSFun__/3(__UniqueInportName__3__)
  Gain/1 -> Subsystem/5(h_1)
  Gain1/1 -> Subsystem/6(h_2)

== system CoupledTanks_original/COUPLED TANKS VR Model1 ==
  Pump : Inport
  Valve Vo1 : Inport  Port=2
  Valve Vt : Inport  Port=3
  Valve Vo2 : Inport  Port=4
  Coupled tanks : M-S-Function  FunctionName=CoupledProngTanks  Parameters=h10 h20  mask{h10=sfcnParam1, h20=sfcnParam2}
      mask prompts: h10 "h1_init"; h20 "h2_init"
      mask Display:
      | port_label('input',1,'Pump');
      | port_label('input',2,'Valve Vo1');
      | port_label('input',3,'Valve Vt');
      | port_label('input',4,'Valve Vo2');
      | port_label('output',1,'Tank 1');
      | port_label('output',2,'Tank 2');
      | port_label('output',3,'q_i');
  Subsystem : Subsystem
  VR Sink : vrlib/VR Sink  InstantiateOnLoad=on  SampleTime=-1  ViewEnable=on  RemoteChange=off  RemoteView=on  FieldsWritten=Valve_t.rotation.4.1.double#Valve_o2.rotation.4.1.double#Valve_o1.rotation.4.1.double#Pump.rotation.4.1.double#water1.scale.3.1.double#water2.scale.3.1.double  WorldFileName=CoupledTanks_VR.WRL  AutoView=off  VideoDimensions=[]  AllowVariableSize=off
  __InputSSForSFun__ : Subsystem
  __OutputSSForSFun__ : Subsystem
  Tank 1 : Outport  OutDataTypeStr=double  PortDimensions=1  SampleTime=[-1 0]
  Tank 2 : Outport  Port=2  OutDataTypeStr=double  PortDimensions=1  SampleTime=[-1 0]
  wires:
  __OutputSSForSFun__/6(q_o2) -> Subsystem/4(q_o2)
  __OutputSSForSFun__/5(q_t) -> Subsystem/3(q_t)
  __OutputSSForSFun__/4(q_o1) -> Subsystem/2(q_o1)
  __OutputSSForSFun__/3(q_i) -> Subsystem/1(q_i)
  Subsystem/2(Q_o2) -> VR Sink/2
  Subsystem/3(Q_o1) -> VR Sink/3
  Subsystem/4(Q_i) -> VR Sink/4
  Subsystem/1(Q_t) -> VR Sink/1
  Subsystem/6(H_2) -> VR Sink/6
  Subsystem/5(H_1) -> VR Sink/5
  __OutputSSForSFun__/2(Tank 2) -> Subsystem/6(h_2), Tank 2/1
  __OutputSSForSFun__/1(Tank 1) -> Tank 1/1, Subsystem/5(h_1)
  __InputSSForSFun__/4(__UniqueOutportName__4__) -> __OutputSSForSFun__/6(__UniqueInportName__6__), Coupled tanks/4
  __InputSSForSFun__/3(__UniqueOutportName__3__) -> __OutputSSForSFun__/5(__UniqueInportName__5__), Coupled tanks/3
  Coupled tanks/2 -> __OutputSSForSFun__/2(__UniqueInportName__2__)
  Coupled tanks/1 -> __OutputSSForSFun__/1(__UniqueInportName__1__)
  __InputSSForSFun__/2(__UniqueOutportName__2__) -> __OutputSSForSFun__/4(__UniqueInportName__4__), Coupled tanks/2
  __InputSSForSFun__/1(__UniqueOutportName__1__) -> Coupled tanks/1
  Valve Vo2/1 -> __InputSSForSFun__/4(Valve Vo2)
  Valve Vt/1 -> __InputSSForSFun__/3(Valve Vt)
  Valve Vo1/1 -> __InputSSForSFun__/2(Valve Vo1)
  Pump/1 -> __InputSSForSFun__/1(Pump)
  Coupled tanks/3 -> __OutputSSForSFun__/3(__UniqueInportName__3__)

== system CoupledTanks_original/COUPLED TANKS VR Model2 ==
  Pump : Inport
  Valve Vo1 : Inport  Port=2
  Valve Vt : Inport  Port=3
  Valve Vo2 : Inport  Port=4
  Coupled tanks : M-S-Function  FunctionName=CoupledProngTanks  Parameters=h10 h20  mask{h10=sfcnParam1, h20=sfcnParam2}
      mask prompts: h10 "h1_init"; h20 "h2_init"
      mask Display:
      | port_label('input',1,'Pump');
      | port_label('input',2,'Valve Vo1');
      | port_label('input',3,'Valve Vt');
      | port_label('input',4,'Valve Vo2');
      | port_label('output',1,'Tank 1');
      | port_label('output',2,'Tank 2');
      | port_label('output',3,'q_i');
  Subsystem : Subsystem
  VR Sink : vrlib/VR Sink  InstantiateOnLoad=on  SampleTime=-1  ViewEnable=on  RemoteChange=off  RemoteView=on  FieldsWritten=Valve_t.rotation.4.1.double#Valve_o2.rotation.4.1.double#Valve_o1.rotation.4.1.double#Pump.rotation.4.1.double#water1.scale.3.1.double#water2.scale.3.1.double  WorldFileName=CoupledTanks_VR.WRL  AutoView=off  VideoDimensions=[]  AllowVariableSize=off
  __InputSSForSFun__ : Subsystem
  __OutputSSForSFun__ : Subsystem
  Tank 1 : Outport  OutDataTypeStr=double  PortDimensions=1  SampleTime=[-1 0]
  Tank 2 : Outport  Port=2  OutDataTypeStr=double  PortDimensions=1  SampleTime=[-1 0]
  wires:
  __OutputSSForSFun__/6(q_o2) -> Subsystem/4(q_o2)
  __OutputSSForSFun__/5(q_t) -> Subsystem/3(q_t)
  __OutputSSForSFun__/4(q_o1) -> Subsystem/2(q_o1)
  __OutputSSForSFun__/3(q_i) -> Subsystem/1(q_i)
  Subsystem/2(Q_o2) -> VR Sink/2
  Subsystem/3(Q_o1) -> VR Sink/3
  Subsystem/4(Q_i) -> VR Sink/4
  Subsystem/1(Q_t) -> VR Sink/1
  Subsystem/6(H_2) -> VR Sink/6
  Subsystem/5(H_1) -> VR Sink/5
  __OutputSSForSFun__/2(Tank 2) -> Subsystem/6(h_2), Tank 2/1
  __OutputSSForSFun__/1(Tank 1) -> Tank 1/1, Subsystem/5(h_1)
  __InputSSForSFun__/4(__UniqueOutportName__4__) -> __OutputSSForSFun__/6(__UniqueInportName__6__), Coupled tanks/4
  __InputSSForSFun__/3(__UniqueOutportName__3__) -> __OutputSSForSFun__/5(__UniqueInportName__5__), Coupled tanks/3
  Coupled tanks/2 -> __OutputSSForSFun__/2(__UniqueInportName__2__)
  Coupled tanks/1 -> __OutputSSForSFun__/1(__UniqueInportName__1__)
  __InputSSForSFun__/2(__UniqueOutportName__2__) -> __OutputSSForSFun__/4(__UniqueInportName__4__), Coupled tanks/2
  __InputSSForSFun__/1(__UniqueOutportName__1__) -> Coupled tanks/1
  Valve Vo2/1 -> __InputSSForSFun__/4(Valve Vo2)
  Valve Vt/1 -> __InputSSForSFun__/3(Valve Vt)
  Valve Vo1/1 -> __InputSSForSFun__/2(Valve Vo1)
  Pump/1 -> __InputSSForSFun__/1(Pump)
  Coupled tanks/3 -> __OutputSSForSFun__/3(__UniqueInportName__3__)

== system CoupledTanks_original/COUPLED TANKS VR Model3 ==
  Pump : Inport
  Valve Vo1 : Inport  Port=2
  Valve Vt : Inport  Port=3
  Valve Vo2 : Inport  Port=4
  Coupled tanks : M-S-Function  FunctionName=CoupledProngTanks  Parameters=h10 h20  mask{h10=sfcnParam1, h20=sfcnParam2}
      mask prompts: h10 "h1_init"; h20 "h2_init"
      mask Display:
      | port_label('input',1,'Pump');
      | port_label('input',2,'Valve Vo1');
      | port_label('input',3,'Valve Vt');
      | port_label('input',4,'Valve Vo2');
      | port_label('output',1,'Tank 1');
      | port_label('output',2,'Tank 2');
      | port_label('output',3,'q_i');
  Subsystem : Subsystem
  VR Sink : vrlib/VR Sink  InstantiateOnLoad=on  SampleTime=-1  ViewEnable=on  RemoteChange=off  RemoteView=on  FieldsWritten=Valve_t.rotation.4.1.double#Valve_o2.rotation.4.1.double#Valve_o1.rotation.4.1.double#Pump.rotation.4.1.double#water1.scale.3.1.double#water2.scale.3.1.double  WorldFileName=CoupledTanks_VR.WRL  AutoView=off  VideoDimensions=[]  AllowVariableSize=off
  __InputSSForSFun__ : Subsystem
  __OutputSSForSFun__ : Subsystem
  Tank 1 : Outport  OutDataTypeStr=double  PortDimensions=1  SampleTime=[-1 0]
  Tank 2 : Outport  Port=2  OutDataTypeStr=double  PortDimensions=1  SampleTime=[-1 0]
  wires:
  __OutputSSForSFun__/6(q_o2) -> Subsystem/4(q_o2)
  __OutputSSForSFun__/5(q_t) -> Subsystem/3(q_t)
  __OutputSSForSFun__/4(q_o1) -> Subsystem/2(q_o1)
  __OutputSSForSFun__/3(q_i) -> Subsystem/1(q_i)
  Subsystem/2(Q_o2) -> VR Sink/2
  Subsystem/3(Q_o1) -> VR Sink/3
  Subsystem/4(Q_i) -> VR Sink/4
  Subsystem/1(Q_t) -> VR Sink/1
  Subsystem/6(H_2) -> VR Sink/6
  Subsystem/5(H_1) -> VR Sink/5
  __OutputSSForSFun__/2(Tank 2) -> Subsystem/6(h_2), Tank 2/1
  __OutputSSForSFun__/1(Tank 1) -> Tank 1/1, Subsystem/5(h_1)
  __InputSSForSFun__/4(__UniqueOutportName__4__) -> __OutputSSForSFun__/6(__UniqueInportName__6__), Coupled tanks/4
  __InputSSForSFun__/3(__UniqueOutportName__3__) -> __OutputSSForSFun__/5(__UniqueInportName__5__), Coupled tanks/3
  Coupled tanks/2 -> __OutputSSForSFun__/2(__UniqueInportName__2__)
  Coupled tanks/1 -> __OutputSSForSFun__/1(__UniqueInportName__1__)
  __InputSSForSFun__/2(__UniqueOutportName__2__) -> __OutputSSForSFun__/4(__UniqueInportName__4__), Coupled tanks/2
  __InputSSForSFun__/1(__UniqueOutportName__1__) -> Coupled tanks/1
  Valve Vo2/1 -> __InputSSForSFun__/4(Valve Vo2)
  Valve Vt/1 -> __InputSSForSFun__/3(Valve Vt)
  Valve Vo1/1 -> __InputSSForSFun__/2(Valve Vo1)
  Pump/1 -> __InputSSForSFun__/1(Pump)
  Coupled tanks/3 -> __OutputSSForSFun__/3(__UniqueInportName__3__)
